simulink model "chapter3_jd"  (R2016b)
settings: Solver=VariableStepAuto  StartTime=0.0  StopTime=10.0  RelTol=1e-3
settings Model: Creator=training-ah  LastModifiedBy=training-ah

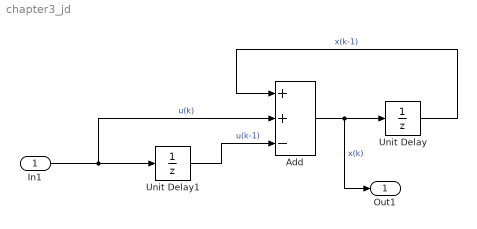
== system chapter3_jd ==
  In1 : Inport
  Add : Sum  Inputs=++-
  Unit Delay : UnitDelay  SampleTime=-1
  Unit Delay1 : UnitDelay  SampleTime=-1
  Out1 : Outport
  wires:
  Add/1 -> Out1/1, Unit Delay/1  "x(k)"
  Unit Delay/1 -> Add/1  "x(k-1)"
  In1/1 -> Add/2, Unit Delay1/1  "u(k)"
  Unit Delay1/1 -> Add/3  "u(k-1)"
